simulink model "simple_robot"  (R2017b)
settings: Solver=FixedStepAuto  StartTime=0.0  StopTime=10.0  FixedStep=0.01  RelTol=1e-3
settings Model: Creator=zhenya  LastModifiedBy=ernst
settings DataIOCC: ExternalInput=[t__, u__]  LoadExternalInput=on  SaveFormat=StructureWithTime

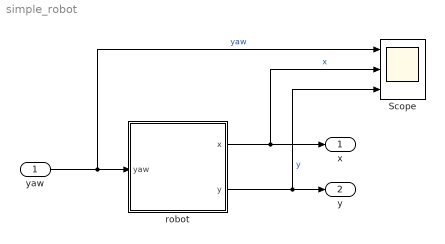
== system simple_robot ==
  yaw : Inport  Interpolate=off
  Scope : Scope  NumInputPorts=3
  robot : Subsystem
  x : Outport
  y : Outport  Port=2
  wires:
  yaw/1 -> Scope/1, robot/1(yaw)  "yaw"
  robot/1(x) -> Scope/2, x/1  "x"
  robot/2(y) -> Scope/3, y/1  "y"

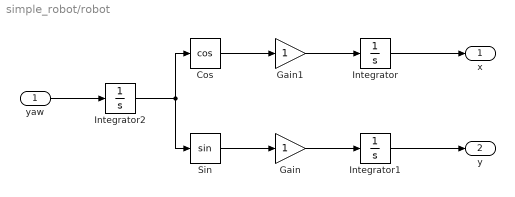
== system simple_robot/robot ==
  yaw : Inport
  Cos : Trigonometry  Operator=cos
  Gain : Gain
  Gain1 : Gain
  Integrator : Integrator
  Integrator1 : Integrator
  Integrator2 : Integrator
  Sin : Trigonometry
  x : Outport
  y : Outport  Port=2
  wires:
  Gain1/1 -> Integrator/1
  Gain/1 -> Integrator1/1
  yaw/1 -> Integrator2/1
  Sin/1 -> Gain/1
  Cos/1 -> Gain1/1
  Integrator/1 -> x/1
  Integrator1/1 -> y/1
  Integrator2/1 -> Cos/1, Sin/1
